simulink model "led_toggle_1Hz_am13x"  (R2025b)
settings: Solver=FixedStepAuto  StartTime=0.0  StopTime=10.0  RelTol=1e-3  EnableMultiTasking=on
settings Model: Creator=a0542960  LastModifiedBy=a1255762
settings OptimizationCC: EnhancedBackFolding=on  PassReuseOutputArgsAs=Individual arguments  ZeroExternalMemoryAtStartup=off  ZeroInternalMemoryAtStartup=off  MaxStackSize=64  OptimizeBlockOrder=speed  DifferentSizesBufferReuse=on  OptimizationCustomize=off  EfficientTunableParamExpr=on
settings DebuggingCC: ParameterTunabilityLossMsg=error
settings HardwareCC: ProdBitPerPointer=32.0  ProdBitPerSizeT=32.0  ProdBitPerPtrDiffT=32.0  ProdLargestAtomicInteger=Long  ProdLargestAtomicFloat=Double  ProdWordSize=32.0  ProdLongLongMode=on  ProdHWDeviceType=ARM Compatible->ARM Cortex
settings SFSimCC: MATLABDynamicMemAlloc=off
settings RTWCC: SystemTargetFile=ert.tlc  HardwareBoard=AM13E230x  TemplateMakefile=ert_default_tmf  Toolchain=TI ARM Clang Compiler AM13x | gmake  BuildConfiguration=Faster Runs  Description=Embedded Coder
settings CodeAppCC: ForceParamTrailComments=on  IgnoreCustomStorageClasses=off  MaxIdLength=256.0  OperatorAnnotations=on  SimulinkDataObjDesc=on  SFDataObjDesc=on  InsertBlockDesc=on
settings ERTTargetCC: ExtModeTransport=3.0  ExtModeStaticAlloc=on  ExtModeMexFile=ext_xcp  ExtModeIntrfLevel=Level2 - Open  InlinedParameterPlacement=Hierarchical  ERTCustomFileTemplate=AM13x_codertarget_file_process.tlc  CodeReplacementLibrary=AM13x_TMU

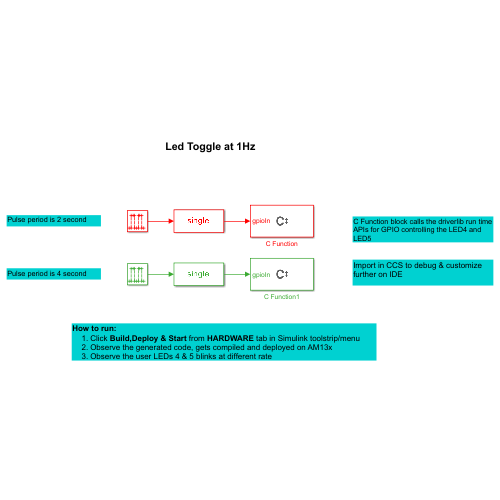
[thumbnail: Simulink's stored preview of the top-level diagram]
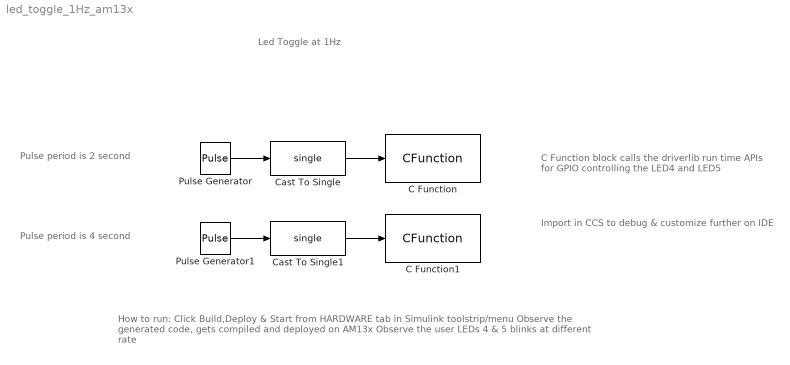
== system led_toggle_1Hz_am13x ==
  note: C Function block calls the driverlib run time APIs for GPIO controlling the LED4 and LED5
  note: Led Toggle at 1Hz
  note: Pulse period is 2 second
  note: Pulse period is 4 second
  note: Import in CCS to debug & customize further on IDE
  note: How to run:
      | Click Build,Deploy & Start from HARDWARE tab in Simulink toolstrip/menu
      | Observe the generated code, gets compiled and deployed on AM13x
      | Observe the user LEDs 4 & 5 blinks at different rate
  C Function : CFunction  CodeGenUsesSimCustomCode=off  CodegenOutputCode=|  CustomHeaderFile=|
      CodegenOutputCode=|
      | if(gpioIn){
      |     DL_GPIO_clearPins(GPIO0, GPIO_LEDS_LED4_PIN);
      | } else{
      |     DL_GPIO_setPins(GPIO0, GPIO_LEDS_LED4_PIN);
      | }
      CustomHeaderFile=|
      | dl_gpio.h
      | hw_memmap.h
      | ti_sdk_dl_config.h
  C Function1 : CFunction  CodeGenUsesSimCustomCode=off  CodegenOutputCode=|  CustomHeaderFile=|
      CodegenOutputCode=|
      | if(gpioIn){
      |     DL_GPIO_clearPins(GPIO1, GPIO_LEDS_LED5_PIN);
      | } else{
      |     DL_GPIO_setPins(GPIO1, GPIO_LEDS_LED5_PIN);
      | }
      CustomHeaderFile=|
      | dl_gpio.h
      | hw_memmap.h
      | ti_sdk_dl_config.h
  Cast To Single : DataTypeConversion  OutDataTypeStr=single  SaturateOnIntegerOverflow=off  RndMeth=Floor
  Cast To Single1 : DataTypeConversion  OutDataTypeStr=single  SaturateOnIntegerOverflow=off  RndMeth=Floor
  Pulse Generator : DiscretePulseGenerator
  Pulse Generator1 : DiscretePulseGenerator  SampleTime=2
  wires:
  Pulse Generator1/1 -> Cast To Single1/1
  Cast To Single1/1 -> C Function1/1
  Pulse Generator/1 -> Cast To Single/1
  Cast To Single/1 -> C Function/1
